simulink model "what2"  (R2021a)
settings: Solver=VariableStepAuto  StartTime=0.0  StopTime=10.0  RelTol=1e-3
model workspace (MAT data in the model file):
  kd = 21212
  kp = 1212
  kpd = 66
  kpp = 12243
settings Model: Creator=rocky  LastModifiedBy=rocky

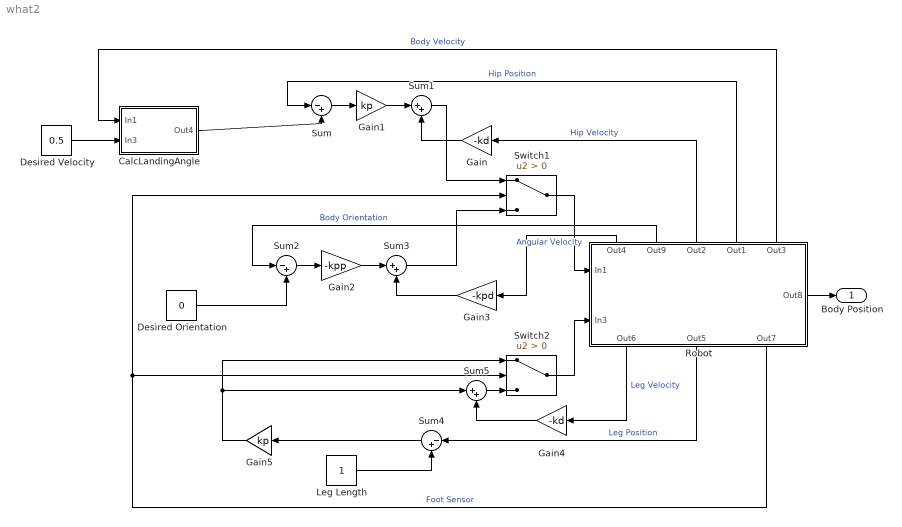
== system what2 ==
  CalcLandingAngle : Subsystem
  Desired Orientation : Constant  Value=0
  Desired Velocity : Constant  Value=0.5
  Gain : Gain  Gain=-kd
  Gain1 : Gain  Gain=kp
  Gain2 : Gain  Gain=-kpp
  Gain3 : Gain  Gain=-kpd
  Gain4 : Gain  Gain=-kd
  Gain5 : Gain  Gain=kp
  Leg Length : Constant
  Robot : Subsystem
      settings: PortSchema="{\"entries\":[{\"content\":{\"sides\":[{\"content\":{\"connectorIds\":[\"In1\",\"In2\"]},\"type\":\"ConnectorPlacement.EquallySpacedRectSide\",\"uuid\":\"9a725299-74fa-49b3-b76c-1a906cc5e7b6\"},{\"content\":{\"connectorIds\":[\"Out1\"],\"side\":\"RIGHT\"},\"type\":\"ConnectorPlacement.EquallySpacedRectSide\",\"uuid\":\"d9382410-c19f-42a1-adce-13800894a608\"},{\"content\":{\"connectorIds\":[\"Out5\",\"Out6\",\"Out7\",\"Out8\",\"Out9\"],\"side\":\"TOP\"},\"type\":\"ConnectorPlacement.EquallySpacedRectSide\",\"uuid\":\"7bb5b47c-24fc-4f05-a8d0-befec55d7818\"},{\"content\":{\"connectorIds\":[\"Out2\",\"Out3\",\"Out4\"],\"side\":\"BOTTOM\"},\"type\":\"ConnectorPlacement.EquallySpacedRectSide\",\"uuid\":\"35ba3e02-b7b8-4fe3-bdfe-00104930865b\"}]},\"type\":\"ConnectorPlacement.EquallySpacedConnector\",\"uuid\":\"f40267b1-a49f-4775-a40f-fa3e87e47f78\"}],\"packageUris\":[\"http://schema.mathworks.com/mf0/Connector/R2020b\"],\"version\":\"1.0\"}"
  Sum : Sum  Inputs=|-+
  Sum1 : Sum  Inputs=|++
  Sum2 : Sum  Inputs=|-+
  Sum3 : Sum  Inputs=|++
  Sum4 : Sum  Inputs=|-+
  Sum5 : Sum  Inputs=|++
  Switch1 : Switch  Criteria=u2 > Threshold
  Switch2 : Switch  Criteria=u2 > Threshold
  Body Position : Outport
  wires:
  CalcLandingAngle/1(Out4) -> Sum/2
  Gain/1 -> Sum1/2
  Sum/1 -> Gain1/1
  Gain1/1 -> Sum1/1
  Sum1/1 -> Switch1/1
  Robot/6(Out9) -> Sum2/1  "Body Orientation"
  Desired Orientation/1 -> Sum2/2
  Sum2/1 -> Gain2/1
  Gain2/1 -> Sum3/1
  Gain3/1 -> Sum3/2
  Sum3/1 -> Switch1/3
  Sum4/1 -> Gain5/1
  Gain4/1 -> Sum5/2
  Sum5/1 -> Switch2/3
  Gain5/1 -> Switch2/1, Sum5/1
  Leg Length/1 -> Sum4/2
  Switch1/1 -> Robot/1(In1)
  Switch2/1 -> Robot/2(In3)
  Robot/8(Out1) -> Sum/1  "Hip Position"
  Robot/7(Out2) -> Gain/1  "Hip Velocity"
  Robot/1(Out8) -> Body Position/1
  Robot/9(Out3) -> CalcLandingAngle/1(In1)  "Body Velocity"
  Robot/5(Out4) -> Gain3/1  "Angular Velocity"
  Robot/4(Out7) -> Switch2/2, Switch1/2  "Foot Sensor"
  Desired Velocity/1 -> CalcLandingAngle/2(In3)
  Robot/2(Out6) -> Gain4/1  "Leg Velocity"
  Robot/3(Out5) -> Sum4/1  "Leg Position"

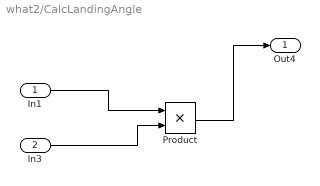
== system what2/CalcLandingAngle ==
  In1 : Inport
  In3 : Inport  Port=2
  Product : Product
  Out4 : Outport
  wires:
  In3/1 -> Product/2
  In1/1 -> Product/1
  Product/1 -> Out4/1

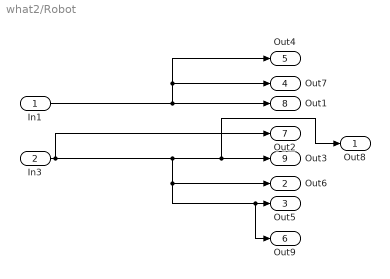
== system what2/Robot ==
  In1 : Inport
  In3 : Inport  Port=2
  Out8 : Outport
  Out6 : Outport  Port=2
  Out5 : Outport  Port=3
  Out7 : Outport  Port=4
  Out4 : Outport  Port=5
  Out9 : Outport  Port=6
  Out2 : Outport  Port=7
  Out1 : Outport  Port=8
  Out3 : Outport  Port=9
  wires:
  In1/1 -> Out7/1, Out4/1, Out1/1
  In3/1 -> Out2/1, Out9/1, Out5/1, Out6/1, Out8/1, Out3/1
